simulink model "Battery_pack"  (R2021b)
settings: Solver=VariableStepAuto  StartTime=0.0  StopTime=500  RelTol=1e-3
undefined symbols (not defined in the file): Ion, Lithium
libraries: spsBatteryLib x10, spsIdealSwitchLib x10, spsSeriesRLCLoadLib x10, spspowerguiLib x1
settings Model: Creator=Ryuk  LastModifiedBy=Ryuk
settings SolverCC: ZeroCrossAlgorithm=Adaptive
settings DebuggingCC: IgnoredZcDiagnostic=none

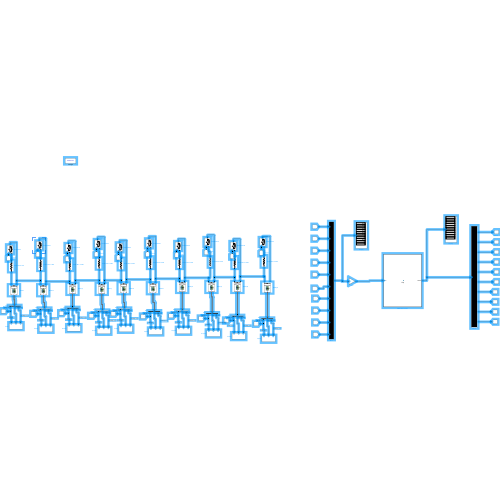
[thumbnail: Simulink's stored preview of the top-level diagram]
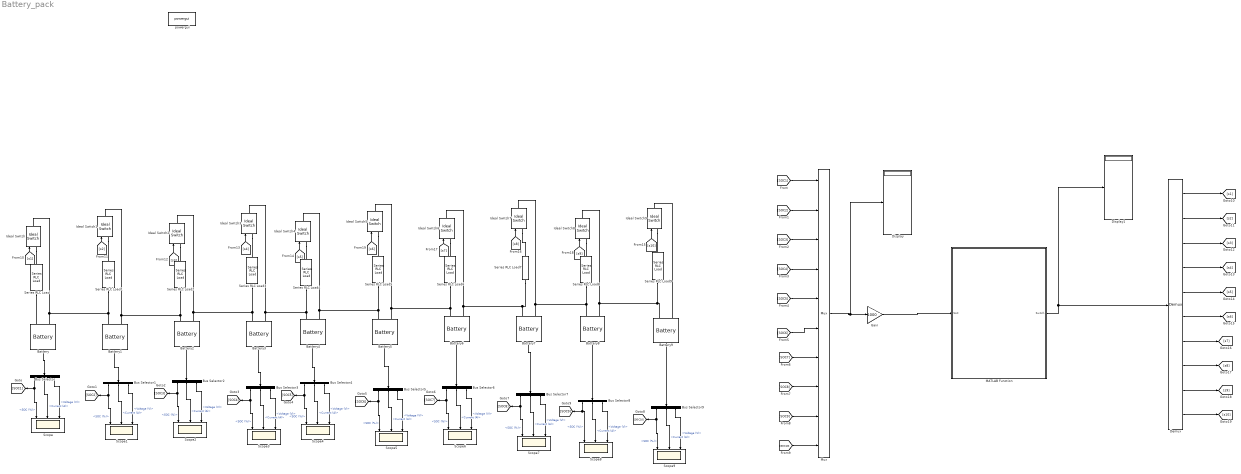
== system Battery_pack ==
  Battery{,1..5,7..9} (9 alike) : spsBatteryLib/Battery  BatType=Lithium-Ion  ShowTempParam=off  ThermalPreset=no  ShowAgeParam=off  NomV=7.2  NomQ=5.4  SOC=100  Batt_Tr=30  PresetModel=on  MaxQ=5.4  MinV=5.4  FullV=8.3807  Dis_rate=2.3478  R=0.013333  Normal_OP=4.8835  expZone="[7.7788      0.2653]"  current=[6.5 13 32.5]  Units=Time  Tci=20  NomT=20  T2=-30  MaxQ2=4.8  FullV2=7.1  Normal_OP2=5.655  expZone2="[6.58           1]"  Rca=0.6  ti=2000  Dp=0  Neq0=0  Tsim=1e6  Ta1=25  Qeol=5.4*0.9  Reol=0.013333*1.2  Char_age=[2.3478, 3]  Dis_age=[2.3478, 10]  N1=1500  N2=10500  N3=1000  N4=1400  Ta2=45  N5=950
  Battery6 : spsBatteryLib/Battery  BatType=Lithium-Ion  ShowTempParam=off  ThermalPreset=no  ShowAgeParam=off  NomV=7.2  NomQ=5.4  SOC=96  Batt_Tr=30  PresetModel=on  MaxQ=5.4  MinV=5.4  FullV=8.3807  Dis_rate=2.3478  R=0.013333  Normal_OP=4.8835  expZone="[7.7788      0.2653]"  current=[6.5 13 32.5]  Units=Time  Tci=20  NomT=20  T2=-30  MaxQ2=4.8  FullV2=7.1  Normal_OP2=5.655  expZone2="[6.58           1]"  Rca=0.6  ti=2000  Dp=0  Neq0=0  Tsim=1e6  Ta1=25  Qeol=5.4*0.9  Reol=0.013333*1.2  Char_age=[2.3478, 3]  Dis_age=[2.3478, 10]  N1=1500  N2=10500  N3=1000  N4=1400  Ta2=45  N5=950
  Bus Selector{,1..9} (10 alike) : BusSelector  OutputSignals=SOC (%),Current (A),Voltage (V)
  Demux : Demux  Outputs=10
  Display : Display
  Display1 : Display
  Gain : Gain  Gain=1000
  Ideal Switch{,1..9} (10 alike) : spsIdealSwitchLib/Ideal Switch  Ron=0.001  Lon=0  IC=0  Rs=1e5  Cs=inf  Measurements=off
  MATLAB Function : MATLAB Function  TreatAsAtomicUnit=on
  Mux : Mux  Inputs=10
  Scope{,1..9} (10 alike) : Scope  NumInputPorts=3
  Series RLC Load : spsSeriesRLCLoadLib/Series RLC Load  LConnTagsString=a  RConnTagsString=__new0  NominalVoltage=3.7  NominalFrequency=.1  ActivePower=1000  InductivePower=0  CapacitivePower=0  Setx0=off  InitialVoltage=0  SetiL0=off  InitialCurrent=0  Measurements=None  LoadType=constant PQ
  Series RLC Load{1..9} (9 alike) : spsSeriesRLCLoadLib/Series RLC Load  LConnTagsString=a  RConnTagsString=__new0  NominalVoltage=3.7  NominalFrequency=.1  ActivePower=1000  InductivePower=0  CapacitivePower=0  Setx0=off  InitialVoltage=0  SetiL0=off  InitialCurrent=0  Measurements=None  LoadType=constant Z
  powergui : spspowerguiLib/powergui  Priority=1  SimulationMode=Continuous  SampleTime=50e-6  frequency=60  Iterations=50  frequencyindice=0  Pbase=100e6  ErrMax=1e-4  UnitsV=kV  UnitsW=MW  buscounter=0  FunctionMessages=off  echomessages=off  EnableUseOfTLC=off  CurrentSourceSwitches=off  DisableSnubberDevices=off  DisableRonSwitches=off  DisableVfSwitches=off  DisplayEquations=off  AutomaticDiscreteSolvers=off  SolverType=Tustin/Backward Euler (TBE)  Interpol=off  ExternalGateDelay=off  methode=off  Ts=100  x0status=blocks  SPID=on  SwTol=0  HookPort=off  NonlinearTolerance=1e-4  nMaxIteration=100  ContinueOnMaxIteration=off  RestoreLinks=warning  ResistiveCurrentMeasurement=off  Frange=[0:2:500]  Ylog=off  Xlog=on  ShowGrid=off  save=off  variable=ZData  structure=0  ZoomFFT=off  StartTime=0.0  cycles=1  DisplayStyle=1  fundamental=60  FreqAxis=off  MaxFrequency=1000  frequencyindicesteady=1  RmsSteady=1  display=off
  wires:
  Bus Selector/3 -> Scope/3  "<Voltage (V)>"
  Bus Selector/2 -> Scope/2  "<Current (A)>"
  Bus Selector/1 -> [SOC1], Scope/1  "<SOC (%)>"
  Battery/1 -> Bus Selector/1
  Battery1/1 -> Bus Selector1/1
  Bus Selector1/1 -> Scope1/1, [SOC2]  "<SOC (%)>"
  Bus Selector1/2 -> Scope1/2  "<Current (A)>"
  Bus Selector1/3 -> Scope1/3  "<Voltage (V)>"
  Bus Selector3/3 -> Scope3/3  "<Voltage (V)>"
  Bus Selector3/2 -> Scope3/2  "<Current (A)>"
  Bus Selector3/1 -> [SOC4], Scope3/1  "<SOC (%)>"
  Battery3/1 -> Bus Selector3/1
  Battery2/1 -> Bus Selector2/1
  Bus Selector2/1 -> Scope2/1, [SOC3]  "<SOC (%)>"
  Bus Selector2/2 -> Scope2/2  "<Current (A)>"
  Bus Selector2/3 -> Scope2/3  "<Voltage (V)>"
  Bus Selector6/3 -> Scope6/3  "<Voltage (V)>"
  Bus Selector6/2 -> Scope6/2  "<Current (A)>"
  Bus Selector6/1 -> [SOC7], Scope6/1  "<SOC (%)>"
  Battery6/1 -> Bus Selector6/1
  Battery7/1 -> Bus Selector7/1
  Bus Selector7/1 -> Scope7/1, [SOC8]  "<SOC (%)>"
  Bus Selector7/2 -> Scope7/2  "<Current (A)>"
  Bus Selector7/3 -> Scope7/3  "<Voltage (V)>"
  Bus Selector5/3 -> Scope5/3  "<Voltage (V)>"
  Bus Selector5/2 -> Scope5/2  "<Current (A)>"
  Bus Selector5/1 -> [SOC6], Scope5/1  "<SOC (%)>"
  Battery5/1 -> Bus Selector5/1
  Battery4/1 -> Bus Selector4/1
  Bus Selector4/1 -> Scope4/1, [SOC5]  "<SOC (%)>"
  Bus Selector4/2 -> Scope4/2  "<Current (A)>"
  Bus Selector4/3 -> Scope4/3  "<Voltage (V)>"
  Bus Selector9/3 -> Scope9/3  "<Voltage (V)>"
  Bus Selector9/2 -> Scope9/2  "<Current (A)>"
  Bus Selector9/1 -> [SOC10], Scope9/1  "<SOC (%)>"
  Battery9/1 -> Bus Selector9/1
  Bus Selector8/1 -> [SOC9], Scope8/1  "<SOC (%)>"
  Bus Selector8/2 -> Scope8/2  "<Current (A)>"
  Bus Selector8/3 -> Scope8/3  "<Voltage (V)>"
  [s1] -> Ideal Switch/1
  [s2] -> Ideal Switch1/1
  [s3] -> Ideal Switch2/1
  [s4] -> Ideal Switch3/1
  [s5] -> Ideal Switch4/1
  [s6] -> Ideal Switch5/1
  [s7] -> Ideal Switch6/1
  [s8] -> Ideal Switch7/1
  [s9] -> Ideal Switch8/1
  [s10] -> Ideal Switch9/1
  MATLAB Function/1(Switch) -> Demux/1, Display1/1
  Battery8/1 -> Bus Selector8/1
  [SOC8] -> Mux/8
  [SOC7] -> Mux/7
  [SOC9] -> Mux/9
  [SOC1] -> Mux/1
  [SOC3] -> Mux/3
  [SOC10] -> Mux/10
  [SOC6] -> Mux/6
  [SOC2] -> Mux/2
  [SOC5] -> Mux/5
  Mux/1 -> Display/1, Gain/1
  [SOC4] -> Mux/4
  Gain/1 -> MATLAB Function/1(SoC)
  Demux/9 -> [s9]
  Demux/2 -> [s2]
  Demux/8 -> [s8]
  Demux/5 -> [s5]
  Demux/7 -> [s7]
  Demux/4 -> [s4]
  Demux/10 -> [s10]
  Demux/1 -> [s1]
  Demux/3 -> [s3]
  Demux/6 -> [s6]
  connections:
  Series RLC Load/LConn1 -- Battery/LConn1
  Ideal Switch/LConn1 -- Series RLC Load/RConn1
  Ideal Switch1/LConn1 -- Series RLC Load1/RConn1
  Ideal Switch/RConn1 -- Battery1/LConn1 -- Series RLC Load1/LConn1 -- Battery/LConn2
  Ideal Switch2/RConn1 -- Battery3/LConn1 -- Series RLC Load3/LConn1 -- Battery2/LConn2
  Ideal Switch3/LConn1 -- Series RLC Load3/RConn1
  Ideal Switch2/LConn1 -- Series RLC Load2/RConn1
  Ideal Switch1/RConn1 -- Battery2/LConn1 -- Series RLC Load2/LConn1 -- Battery1/LConn2
  Ideal Switch5/RConn1 -- Battery6/LConn1 -- Series RLC Load6/LConn1 -- Battery5/LConn2
  Ideal Switch6/LConn1 -- Series RLC Load6/RConn1
  Ideal Switch6/RConn1 -- Battery7/LConn1 -- Series RLC Load7/LConn1 -- Battery6/LConn2
  Ideal Switch4/RConn1 -- Battery5/LConn1 -- Series RLC Load5/LConn1 -- Battery4/LConn2
  Ideal Switch5/LConn1 -- Series RLC Load5/RConn1
  Ideal Switch7/LConn1 -- Series RLC Load7/RConn1
  Ideal Switch4/LConn1 -- Series RLC Load4/RConn1
  Ideal Switch3/RConn1 -- Series RLC Load4/LConn1 -- Battery4/LConn1 -- Battery3/LConn2
  Battery9/LConn2 -- Ideal Switch9/RConn1
  Ideal Switch8/LConn1 -- Series RLC Load8/RConn1
  Ideal Switch9/LConn1 -- Series RLC Load9/RConn1
  Ideal Switch8/RConn1 -- Battery8/LConn2 -- Battery9/LConn1 -- Series RLC Load9/LConn1
  Ideal Switch7/RConn1 -- Battery8/LConn1 -- Series RLC Load8/LConn1 -- Battery7/LConn2

== matlab function Battery_pack/MATLAB Function ==
  data: SoC input; Switch output
function Switch =  Cmpr(SoC)

Switch=  zeros (10,1); 

[Socn, indx]= sort(SoC,"descend");

t=Socn(10);
index= indx(10);
for i=1:9

    if(i==index)
        continue;
    end

    if(Socn(9)<t|| Socn(9)==t)
        break;
    end

    if(Socn(i)>t)
        Switch(indx(i))=1;
        
    end
end
